simulink model "Newton_Euler_Translational_Motion"  (R2018a)
settings: Solver=VariableStepAuto  StartTime=0.0  StopTime=10.0  RelTol=1e-3
libraries: simulink_extras x2
settings Model: Creator=Ibrahim  LastModifiedBy=Ibrahim

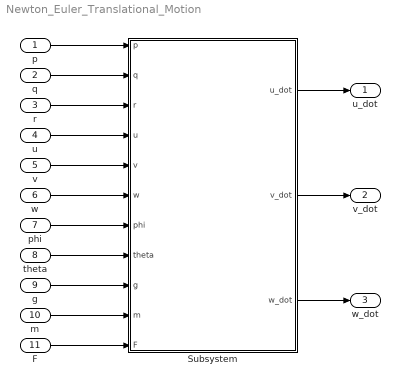
== system Newton_Euler_Translational_Motion ==
  p : Inport
  q : Inport  Port=2
  r : Inport  Port=3
  u : Inport  Port=4
  v : Inport  Port=5
  w : Inport  Port=6
  phi : Inport  Port=7
  theta : Inport  Port=8
  g : Inport  Port=9
  m : Inport  Port=10
  F : Inport  Port=11
  Subsystem : Subsystem
  u_dot : Outport
  v_dot : Outport  Port=2
  w_dot : Outport  Port=3
  wires:
  p/1 -> Subsystem/1(p)
  q/1 -> Subsystem/2(q)
  r/1 -> Subsystem/3(r)
  u/1 -> Subsystem/4(u)
  v/1 -> Subsystem/5(v)
  w/1 -> Subsystem/6(w)
  phi/1 -> Subsystem/7(phi)
  theta/1 -> Subsystem/8(theta)
  g/1 -> Subsystem/9(g)
  m/1 -> Subsystem/10(m)
  F/1 -> Subsystem/11(F)
  Subsystem/1(u_dot) -> u_dot/1
  Subsystem/2(v_dot) -> v_dot/1
  Subsystem/3(w_dot) -> w_dot/1

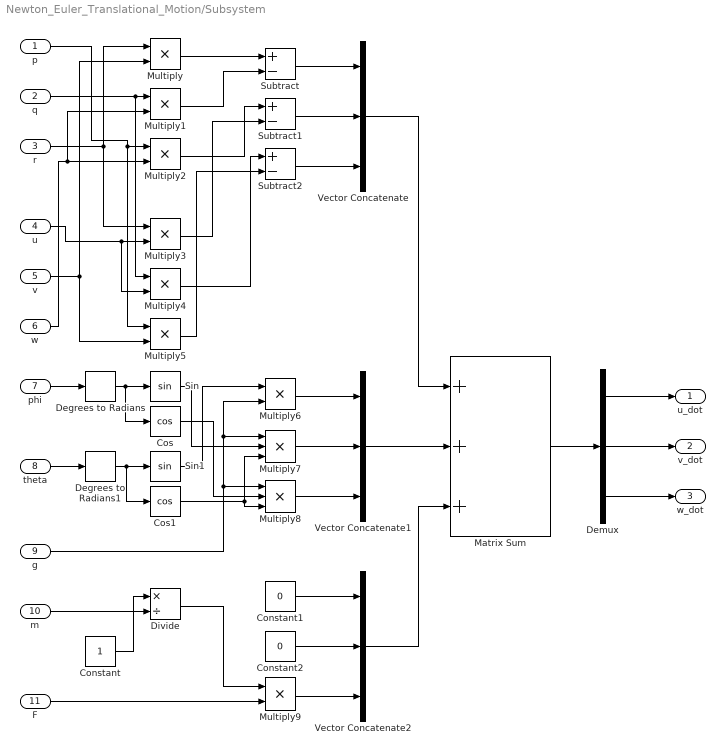
== system Newton_Euler_Translational_Motion/Subsystem ==
  p : Inport
  q : Inport  Port=2
  r : Inport  Port=3
  u : Inport  Port=4
  v : Inport  Port=5
  w : Inport  Port=6
  phi : Inport  Port=7
  theta : Inport  Port=8
  g : Inport  Port=9
  m : Inport  Port=10
  F : Inport  Port=11
  Constant : Constant
  Constant1 : Constant  Value=0
  Constant2 : Constant  Value=0
  Cos : Trigonometry  Operator=cos
  Cos1 : Trigonometry  Operator=cos
  Degrees to Radians : simulink_extras/Transformations/Degrees to Radians
  Degrees to Radians1 : simulink_extras/Transformations/Degrees to Radians
  Demux : Demux  Outputs=3
  Divide : Product  Inputs=*/
  Matrix Sum : Sum  Inputs=+++
  Multiply{,1..6,9} (8 alike) : Product
  Multiply7 : Product  Inputs=3
  Multiply8 : Product  Inputs=3
  Sin : Trigonometry
  Sin1 : Trigonometry
  Subtract : Sum  Inputs=+-
  Subtract1 : Sum  Inputs=+-
  Subtract2 : Sum  Inputs=+-
  Vector Concatenate : Concatenate  NumInputs=3
  Vector Concatenate1 : Concatenate  NumInputs=3
  Vector Concatenate2 : Concatenate  NumInputs=3
  u_dot : Outport
  v_dot : Outport  Port=2
  w_dot : Outport  Port=3
  wires:
  Constant/1 -> Divide/1
  Multiply7/1 -> Vector Concatenate1/2
  Multiply5/1 -> Subtract2/2
  p/1 -> Multiply5/1, Multiply2/1
  Multiply6/1 -> Vector Concatenate1/1
  u/1 -> Multiply3/2, Multiply4/2
  Degrees to Radians1/1 -> Cos1/1, Sin1/1
  theta/1 -> Degrees to Radians1/1
  Demux/1 -> u_dot/1
  Sin/1 -> Multiply7/2
  Vector Concatenate2/1 -> Matrix Sum/3
  Multiply2/1 -> Subtract1/1
  Vector Concatenate/1 -> Matrix Sum/1
  q/1 -> Multiply4/1, Multiply1/1
  Multiply3/1 -> Subtract1/2
  g/1 -> Multiply8/1, Multiply7/1, Multiply6/2
  Sin1/1 -> Multiply6/1
  Constant1/1 -> Vector Concatenate2/1
  Multiply4/1 -> Subtract2/1
  Multiply8/1 -> Vector Concatenate1/3
  phi/1 -> Degrees to Radians/1
  Constant2/1 -> Vector Concatenate2/2
  r/1 -> Multiply3/1, Multiply/1
  Cos/1 -> Multiply8/2
  Subtract2/1 -> Vector Concatenate/3
  Demux/2 -> v_dot/1
  Degrees to Radians/1 -> Cos/1, Sin/1
  Multiply9/1 -> Vector Concatenate2/3
  Subtract/1 -> Vector Concatenate/1
  Multiply/1 -> Subtract/1
  Divide/1 -> Multiply9/1
  Cos1/1 -> Multiply8/3, Multiply7/3
  v/1 -> Multiply5/2, Multiply/2
  Vector Concatenate1/1 -> Matrix Sum/2
  m/1 -> Divide/2
  F/1 -> Multiply9/2
  Subtract1/1 -> Vector Concatenate/2
  w/1 -> Multiply2/2, Multiply1/2
  Multiply1/1 -> Subtract/2
  Matrix Sum/1 -> Demux/1
  Demux/3 -> w_dot/1
